simulink model "suspension_controller_road_condition2"  (R2020a)
settings: Solver=VariableStepAuto  StartTime=0.0  StopTime=10.0  MaxStep=0.1  RelTol=1e-3
values from neighbouring files (symbols this model uses):
  cfs = 1290    [half_car_parameter.m]
  cft = 1000    [half_car_parameter.m]
  crs = 1620    [half_car_parameter.m]
  crt = 1000    [half_car_parameter.m]
  iyy = 2460    [half_car_parameter.m]
  kfs = 19960    [half_car_parameter.m]
  kft = 175500    [half_car_parameter.m]
  krs = 17500    [half_car_parameter.m]
  krt = 175500    [half_car_parameter.m]
  lf = 2.3    [half_car_parameter.m]
  lr = 2.3    [half_car_parameter.m]
  mc = 700    [half_car_parameter.m]
  mf = 40    [half_car_parameter.m]
  mr = 35.5    [half_car_parameter.m]
(part 1 of 2)
settings Model: Creator=USER  LastModifiedBy=USER

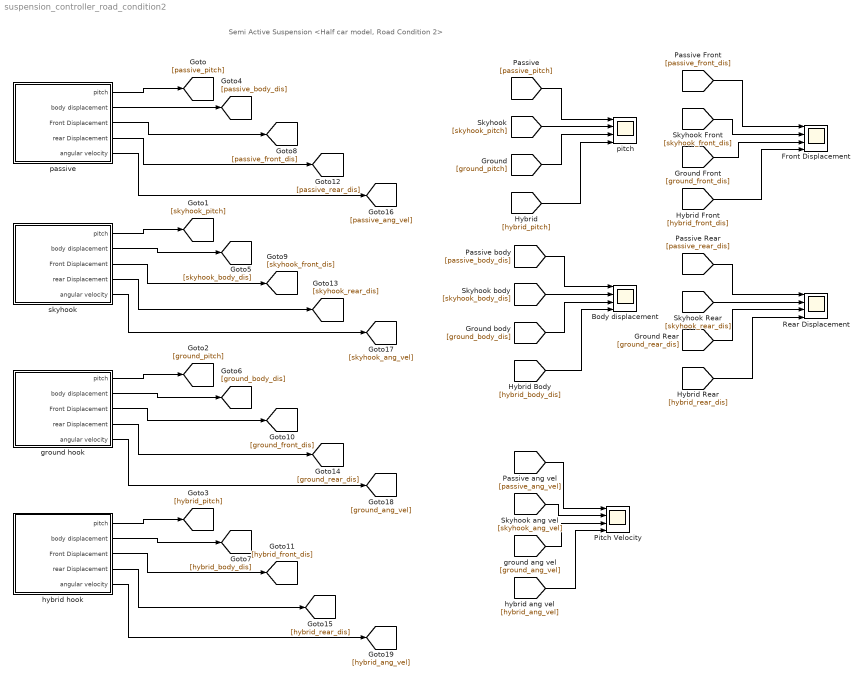
== system suspension_controller_road_condition2 ==
  note: Semi Active Suspension <Half car model, Road Condition 2>
  Body displacement : Scope  NumInputPorts=4
  Front Displacement : Scope  NumInputPorts=4
  Pitch Velocity : Scope  NumInputPorts=4
  Rear Displacement : Scope  NumInputPorts=4
  ground hook : Subsystem
  hybrid hook : Subsystem
  passive : Subsystem
  pitch : Scope  NumInputPorts=4
  skyhook : Subsystem
  wires:
  passive/1(pitch) -> [passive_pitch]
  skyhook/1(pitch) -> [skyhook_pitch]
  ground hook/1(pitch) -> [ground_pitch]
  hybrid hook/1(pitch) -> [hybrid_pitch]
  passive/2(body displacement) -> [passive_body_dis]
  skyhook/2(body displacement) -> [skyhook_body_dis]
  ground hook/2(body displacement) -> [ground_body_dis]
  hybrid hook/2(body displacement) -> [hybrid_body_dis]
  [passive_pitch] -> pitch/1
  [skyhook_pitch] -> pitch/2
  [ground_pitch] -> pitch/3
  [hybrid_pitch] -> pitch/4
  [passive_body_dis] -> Body displacement/1
  [skyhook_body_dis] -> Body displacement/2
  [ground_body_dis] -> Body displacement/3
  [hybrid_body_dis] -> Body displacement/4
  passive/3(Front Displacement) -> [passive_front_dis]
  skyhook/3(Front Displacement) -> [skyhook_front_dis]
  ground hook/3(Front Displacement) -> [ground_front_dis]
  hybrid hook/3(Front Displacement) -> [hybrid_front_dis]
  [passive_front_dis] -> Front Displacement/1
  [skyhook_front_dis] -> Front Displacement/2
  [ground_front_dis] -> Front Displacement/3
  [hybrid_front_dis] -> Front Displacement/4
  passive/4(rear Displacement) -> [passive_rear_dis]
  skyhook/4(rear Displacement) -> [skyhook_rear_dis]
  ground hook/4(rear Displacement) -> [ground_rear_dis]
  hybrid hook/4(rear Displacement) -> [hybrid_rear_dis]
  [hybrid_rear_dis] -> Rear Displacement/4
  [passive_rear_dis] -> Rear Displacement/1
  [ground_rear_dis] -> Rear Displacement/3
  [skyhook_rear_dis] -> Rear Displacement/2
  passive/5(angular velocity) -> [passive_ang_vel]
  skyhook/5(angular velocity) -> [skyhook_ang_vel]
  ground hook/5(angular velocity) -> [ground_ang_vel]
  hybrid hook/5(angular velocity) -> [hybrid_ang_vel]
  [passive_ang_vel] -> Pitch Velocity/1
  [skyhook_ang_vel] -> Pitch Velocity/2
  [ground_ang_vel] -> Pitch Velocity/3
  [hybrid_ang_vel] -> Pitch Velocity/4

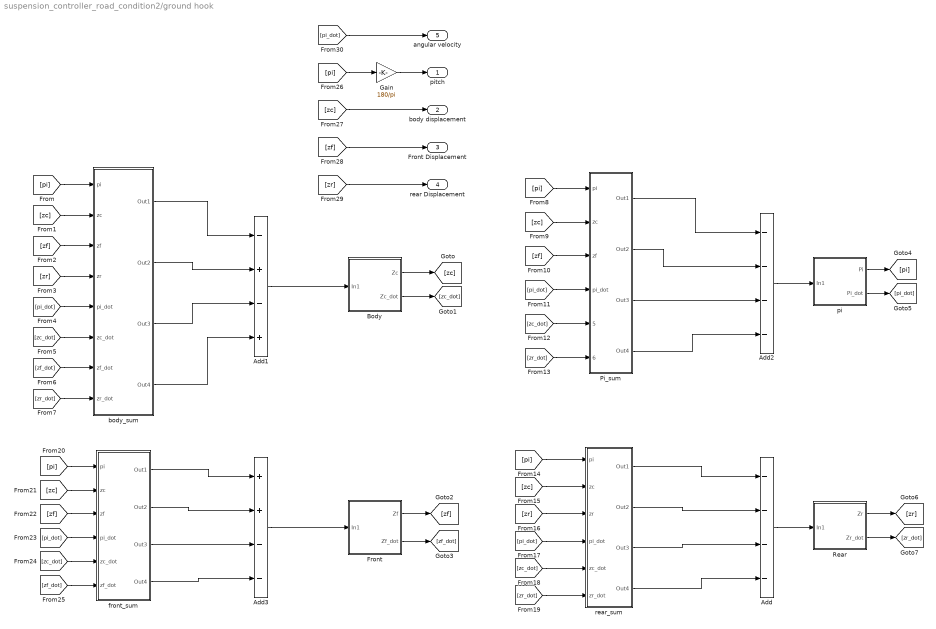
== system suspension_controller_road_condition2/ground hook ==
  Add : Sum  Inputs=----
  Add1 : Sum  Inputs=-+-+
  Add2 : Sum  Inputs=----
  Add3 : Sum  Inputs=++--
  Body : Subsystem
  Front : Subsystem
  Gain : Gain  Gain=180/pi
  Pi_sum : Subsystem
  Rear : Subsystem
  body_sum : Subsystem
  front_sum : Subsystem
  pi : Subsystem
  rear_sum : Subsystem
  pitch : Outport
  body displacement : Outport  Port=2
  Front Displacement : Outport  Port=3
  rear Displacement : Outport  Port=4
  angular velocity : Outport  Port=5
  wires:
  Rear/2(Zr_dot) -> [zr_dot]
  [zc_dot] -> front_sum/5(zc_dot)
  [zr] -> body_sum/4(zr)
  [zr_dot] -> rear_sum/6(zr_dot)
  [pi_dot] -> body_sum/5(pi_dot)
  body_sum/3(Out3) -> Add1/3
  [zr] -> rear_sum/3(zr)
  [pi] -> front_sum/1(pi)
  [zc_dot] -> body_sum/6(zc_dot)
  [zr_dot] -> body_sum/8(zr_dot)
  Front/1(Zf) -> [zf]
  [zf_dot] -> body_sum/7(zf_dot)
  rear_sum/3(Out3) -> Add/3
  body_sum/1(Out1) -> Add1/1
  rear_sum/4(Out4) -> Add/4
  [pi_dot] -> rear_sum/4(pi_dot)
  rear_sum/2(Out2) -> Add/2
  [zc] -> rear_sum/2(zc)
  [pi] -> rear_sum/1(pi)
  Add3/1 -> Front/1(In1)
  rear_sum/1(Out1) -> Add/1
  front_sum/3(Out3) -> Add3/3
  front_sum/4(Out4) -> Add3/4
  front_sum/1(Out1) -> Add3/1
  body_sum/4(Out4) -> Add1/4
  body_sum/2(Out2) -> Add1/2
  Body/1(Zc) -> [zc]
  front_sum/2(Out2) -> Add3/2
  Body/2(Zc_dot) -> [zc_dot]
  Add1/1 -> Body/1(In1)
  Add/1 -> Rear/1(In1)
  [zc] -> body_sum/2(zc)
  [zf] -> body_sum/3(zf)
  [zc_dot] -> rear_sum/5(zc_dot)
  [zf_dot] -> front_sum/6(zf_dot)
  Front/2(Zf_dot) -> [zf_dot]
  Rear/1(Zr) -> [zr]
  [pi] -> body_sum/1(pi)
  [pi_dot] -> front_sum/4(pi_dot)
  [zf] -> front_sum/3(zf)
  [zc] -> front_sum/2(zc)
  Pi_sum/2(Out2) -> Add2/2
  [zc_dot] -> Pi_sum/5(zc_dot)
  [zf] -> Pi_sum/3(zf)
  Pi_sum/4(Out4) -> Add2/4
  [pi] -> Pi_sum/1(pi)
  Pi_sum/3(Out3) -> Add2/3
  [zr_dot] -> Pi_sum/6(zr_dot)
  pi/2(Pi_dot) -> [pi_dot]
  [zc] -> Pi_sum/2(zc)
  [pi_dot] -> Pi_sum/4(pi_dot)
  Pi_sum/1(Out1) -> Add2/1
  pi/1(Pi) -> [pi]
  Add2/1 -> pi/1(In1)
  Gain/1 -> pitch/1
  [pi] -> Gain/1
  [zf] -> Front Displacement/1
  [pi_dot] -> angular velocity/1
  [zr] -> rear Displacement/1
  [zc] -> body displacement/1

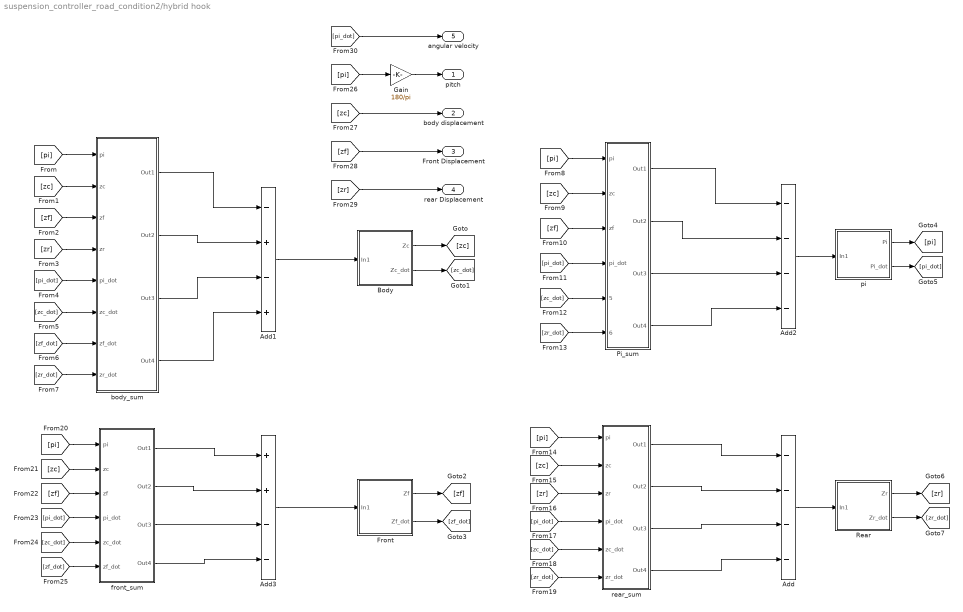
== system suspension_controller_road_condition2/hybrid hook ==
  Add : Sum  Inputs=----
  Add1 : Sum  Inputs=-+-+
  Add2 : Sum  Inputs=----
  Add3 : Sum  Inputs=++--
  Body : Subsystem
  Front : Subsystem
  Gain : Gain  Gain=180/pi
  Pi_sum : Subsystem
  Rear : Subsystem
  body_sum : Subsystem
  front_sum : Subsystem
  pi : Subsystem
  rear_sum : Subsystem
  pitch : Outport
  body displacement : Outport  Port=2
  Front Displacement : Outport  Port=3
  rear Displacement : Outport  Port=4
  angular velocity : Outport  Port=5
  wires:
  Rear/2(Zr_dot) -> [zr_dot]
  [zc_dot] -> front_sum/5(zc_dot)
  [zr] -> body_sum/4(zr)
  [zr_dot] -> rear_sum/6(zr_dot)
  [pi_dot] -> body_sum/5(pi_dot)
  body_sum/3(Out3) -> Add1/3
  [zr] -> rear_sum/3(zr)
  [pi] -> front_sum/1(pi)
  [zc_dot] -> body_sum/6(zc_dot)
  [zr_dot] -> body_sum/8(zr_dot)
  Front/1(Zf) -> [zf]
  [zf_dot] -> body_sum/7(zf_dot)
  rear_sum/3(Out3) -> Add/3
  body_sum/1(Out1) -> Add1/1
  rear_sum/4(Out4) -> Add/4
  [pi_dot] -> rear_sum/4(pi_dot)
  rear_sum/2(Out2) -> Add/2
  [zc] -> rear_sum/2(zc)
  [pi] -> rear_sum/1(pi)
  Add3/1 -> Front/1(In1)
  rear_sum/1(Out1) -> Add/1
  front_sum/3(Out3) -> Add3/3
  front_sum/4(Out4) -> Add3/4
  front_sum/1(Out1) -> Add3/1
  body_sum/4(Out4) -> Add1/4
  body_sum/2(Out2) -> Add1/2
  Body/1(Zc) -> [zc]
  front_sum/2(Out2) -> Add3/2
  Body/2(Zc_dot) -> [zc_dot]
  Add1/1 -> Body/1(In1)
  Add/1 -> Rear/1(In1)
  [zc] -> body_sum/2(zc)
  [zf] -> body_sum/3(zf)
  [zc_dot] -> rear_sum/5(zc_dot)
  [zf_dot] -> front_sum/6(zf_dot)
  Front/2(Zf_dot) -> [zf_dot]
  Rear/1(Zr) -> [zr]
  [pi] -> body_sum/1(pi)
  [pi_dot] -> front_sum/4(pi_dot)
  [zf] -> front_sum/3(zf)
  [zc] -> front_sum/2(zc)
  Pi_sum/2(Out2) -> Add2/2
  [zc_dot] -> Pi_sum/5(zc_dot)
  [zf] -> Pi_sum/3(zf)
  Pi_sum/4(Out4) -> Add2/4
  [pi] -> Pi_sum/1(pi)
  Pi_sum/3(Out3) -> Add2/3
  [zr_dot] -> Pi_sum/6(zr_dot)
  pi/2(Pi_dot) -> [pi_dot]
  [zc] -> Pi_sum/2(zc)
  [pi_dot] -> Pi_sum/4(pi_dot)
  Pi_sum/1(Out1) -> Add2/1
  pi/1(Pi) -> [pi]
  Add2/1 -> pi/1(In1)
  Gain/1 -> pitch/1
  [pi] -> Gain/1
  [zf] -> Front Displacement/1
  [pi_dot] -> angular velocity/1
  [zr] -> rear Displacement/1
  [zc] -> body displacement/1

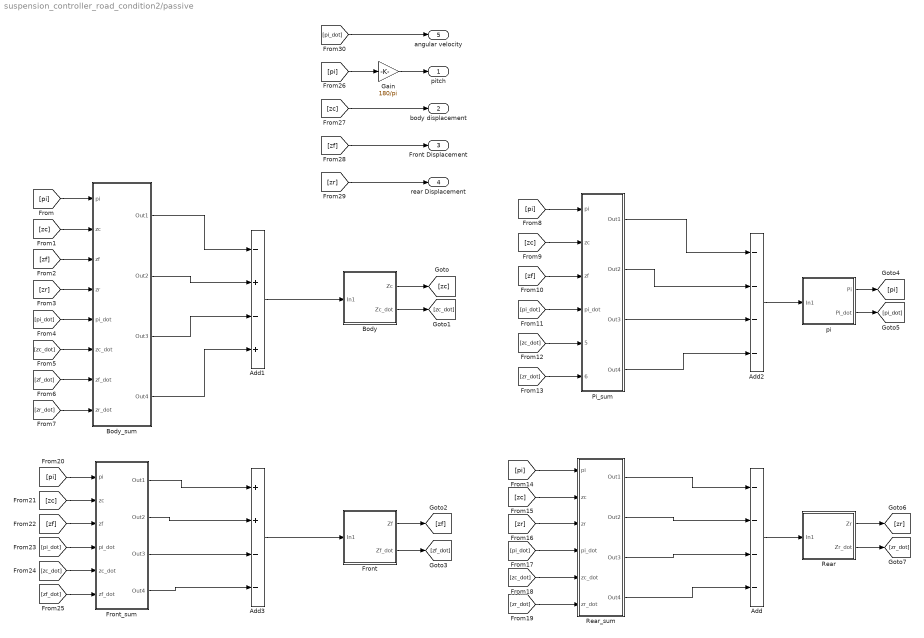
== system suspension_controller_road_condition2/passive ==
  Add : Sum  Inputs=----
  Add1 : Sum  Inputs=-+-+
  Add2 : Sum  Inputs=----
  Add3 : Sum  Inputs=++--
  Body : Subsystem
  Body_sum : Subsystem
  Front : Subsystem
  Front_sum : Subsystem
  Gain : Gain  Gain=180/pi
  Pi_sum : Subsystem
  Rear : Subsystem
  Rear_sum : Subsystem
  pi : Subsystem
  pitch : Outport
  body displacement : Outport  Port=2
  Front Displacement : Outport  Port=3
  rear Displacement : Outport  Port=4
  angular velocity : Outport  Port=5
  wires:
  [zc] -> body displacement/1
  Rear/2(Zr_dot) -> [zr_dot]
  [zc_dot] -> Front_sum/5(zc_dot)
  [zr] -> Body_sum/4(zr)
  [zr_dot] -> Rear_sum/6(zr_dot)
  [pi_dot] -> Body_sum/5(pi_dot)
  Body_sum/3(Out3) -> Add1/3
  [zr] -> Rear_sum/3(zr)
  [pi] -> Front_sum/1(pi)
  [zc_dot] -> Body_sum/6(zc_dot)
  [zr_dot] -> Body_sum/8(zr_dot)
  Front/1(Zf) -> [zf]
  Pi_sum/3(Out3) -> Add2/3
  Pi_sum/2(Out2) -> Add2/2
  [pi] -> Gain/1
  pi/1(Pi) -> [pi]
  [zf_dot] -> Body_sum/7(zf_dot)
  Rear_sum/3(Out3) -> Add/3
  Body_sum/1(Out1) -> Add1/1
  Rear_sum/4(Out4) -> Add/4
  [zc_dot] -> Pi_sum/5(zc_dot)
  [pi_dot] -> Rear_sum/4(pi_dot)
  [zr_dot] -> Pi_sum/6(zr_dot)
  Rear_sum/2(Out2) -> Add/2
  [zc] -> Pi_sum/2(zc)
  [zc] -> Rear_sum/2(zc)
  [pi] -> Rear_sum/1(pi)
  Add3/1 -> Front/1(In1)
  Rear_sum/1(Out1) -> Add/1
  Front_sum/3(Out3) -> Add3/3
  Front_sum/4(Out4) -> Add3/4
  [pi] -> Pi_sum/1(pi)
  Add2/1 -> pi/1(In1)
  Front_sum/1(Out1) -> Add3/1
  Pi_sum/4(Out4) -> Add2/4
  Pi_sum/1(Out1) -> Add2/1
  Body_sum/4(Out4) -> Add1/4
  Body_sum/2(Out2) -> Add1/2
  Body/1(Zc) -> [zc]
  [pi_dot] -> Pi_sum/4(pi_dot)
  Front_sum/2(Out2) -> Add3/2
  Body/2(Zc_dot) -> [zc_dot]
  Add1/1 -> Body/1(In1)
  Add/1 -> Rear/1(In1)
  pi/2(Pi_dot) -> [pi_dot]
  [zc] -> Body_sum/2(zc)
  [zf] -> Body_sum/3(zf)
  [zc_dot] -> Rear_sum/5(zc_dot)
  [zf_dot] -> Front_sum/6(zf_dot)
  Front/2(Zf_dot) -> [zf_dot]
  Rear/1(Zr) -> [zr]
  [pi] -> Body_sum/1(pi)
  [pi_dot] -> Front_sum/4(pi_dot)
  [zf] -> Front_sum/3(zf)
  [zf] -> Pi_sum/3(zf)
  [zc] -> Front_sum/2(zc)
  Gain/1 -> pitch/1
  [zf] -> Front Displacement/1
  [zr] -> rear Displacement/1
  [pi_dot] -> angular velocity/1

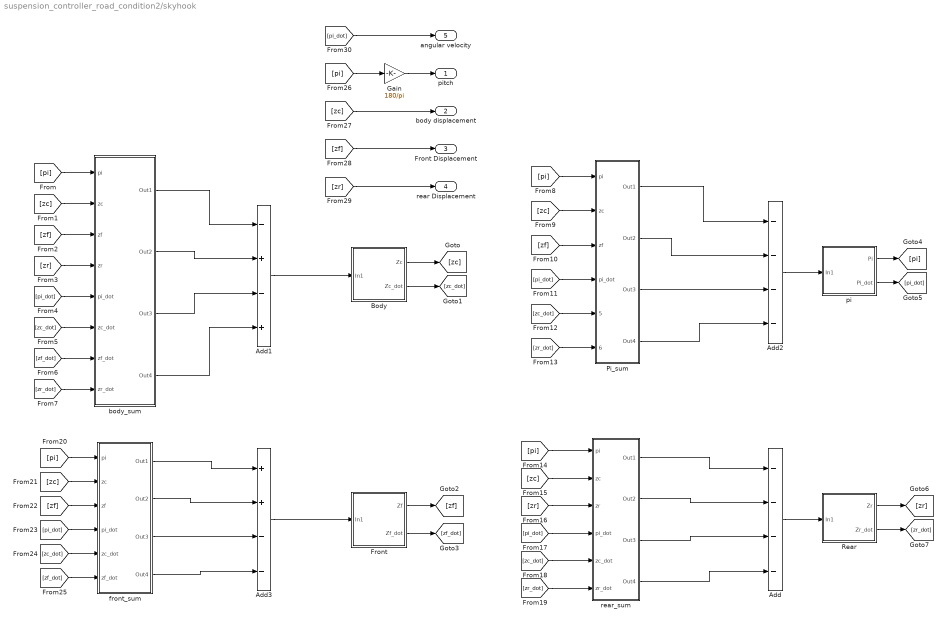
== system suspension_controller_road_condition2/skyhook ==
  Add : Sum  Inputs=----
  Add1 : Sum  Inputs=-+-+
  Add2 : Sum  Inputs=----
  Add3 : Sum  Inputs=++--
  Body : Subsystem
  Front : Subsystem
  Gain : Gain  Gain=180/pi
  Pi_sum : Subsystem
  Rear : Subsystem
  body_sum : Subsystem
  front_sum : Subsystem
  pi : Subsystem
  rear_sum : Subsystem
  pitch : Outport
  body displacement : Outport  Port=2
  Front Displacement : Outport  Port=3
  rear Displacement : Outport  Port=4
  angular velocity : Outport  Port=5
  wires:
  Rear/2(Zr_dot) -> [zr_dot]
  [zc_dot] -> front_sum/5(zc_dot)
  [zr] -> body_sum/4(zr)
  [zr_dot] -> rear_sum/6(zr_dot)
  [pi_dot] -> body_sum/5(pi_dot)
  body_sum/3(Out3) -> Add1/3
  [zr] -> rear_sum/3(zr)
  [pi] -> front_sum/1(pi)
  [zc_dot] -> body_sum/6(zc_dot)
  [zr_dot] -> body_sum/8(zr_dot)
  Front/1(Zf) -> [zf]
  [zf_dot] -> body_sum/7(zf_dot)
  rear_sum/3(Out3) -> Add/3
  body_sum/1(Out1) -> Add1/1
  rear_sum/4(Out4) -> Add/4
  [pi_dot] -> rear_sum/4(pi_dot)
  rear_sum/2(Out2) -> Add/2
  [zc] -> rear_sum/2(zc)
  [pi] -> rear_sum/1(pi)
  Add3/1 -> Front/1(In1)
  rear_sum/1(Out1) -> Add/1
  front_sum/3(Out3) -> Add3/3
  front_sum/4(Out4) -> Add3/4
  front_sum/1(Out1) -> Add3/1
  body_sum/4(Out4) -> Add1/4
  body_sum/2(Out2) -> Add1/2
  Body/1(Zc) -> [zc]
  front_sum/2(Out2) -> Add3/2
  Body/2(Zc_dot) -> [zc_dot]
  Add1/1 -> Body/1(In1)
  Add/1 -> Rear/1(In1)
  [zc] -> body_sum/2(zc)
  [zf] -> body_sum/3(zf)
  [zc_dot] -> rear_sum/5(zc_dot)
  [zf_dot] -> front_sum/6(zf_dot)
  Front/2(Zf_dot) -> [zf_dot]
  Rear/1(Zr) -> [zr]
  [pi] -> body_sum/1(pi)
  [pi_dot] -> front_sum/4(pi_dot)
  [zf] -> front_sum/3(zf)
  [zc] -> front_sum/2(zc)
  Pi_sum/2(Out2) -> Add2/2
  [zc_dot] -> Pi_sum/5(zc_dot)
  [zf] -> Pi_sum/3(zf)
  Pi_sum/4(Out4) -> Add2/4
  [pi] -> Pi_sum/1(pi)
  Pi_sum/3(Out3) -> Add2/3
  [zr_dot] -> Pi_sum/6(zr_dot)
  pi/2(Pi_dot) -> [pi_dot]
  [zc] -> Pi_sum/2(zc)
  [pi_dot] -> Pi_sum/4(pi_dot)
  Pi_sum/1(Out1) -> Add2/1
  pi/1(Pi) -> [pi]
  Add2/1 -> pi/1(In1)
  Gain/1 -> pitch/1
  [pi] -> Gain/1
  [zf] -> Front Displacement/1
  [pi_dot] -> angular velocity/1
  [zr] -> rear Displacement/1
  [zc] -> body displacement/1

== system suspension_controller_road_condition2/ground hook/Body ==
  In1 : Inport
  Gain1 : Gain  Gain=1/mc
  zc : Integrator
  zc_dot : Integrator
  Zc : Outport
  Zc_dot : Outport  Port=2
  wires:
  Gain1/1 -> zc_dot/1  "zc_ddot"
  zc_dot/1 -> Zc_dot/1, zc/1
  In1/1 -> Gain1/1
  zc/1 -> Zc/1

== system suspension_controller_road_condition2/ground hook/Front ==
  In1 : Inport
  Gain2 : Gain  Gain=1/mf
  zf : Integrator
  zf_dot : Integrator
  Zf : Outport
  Zf_dot : Outport  Port=2
  wires:
  In1/1 -> Gain2/1
  zf_dot/1 -> Zf_dot/1, zf/1
  Gain2/1 -> zf_dot/1  "zf_ddot"
  zf/1 -> Zf/1

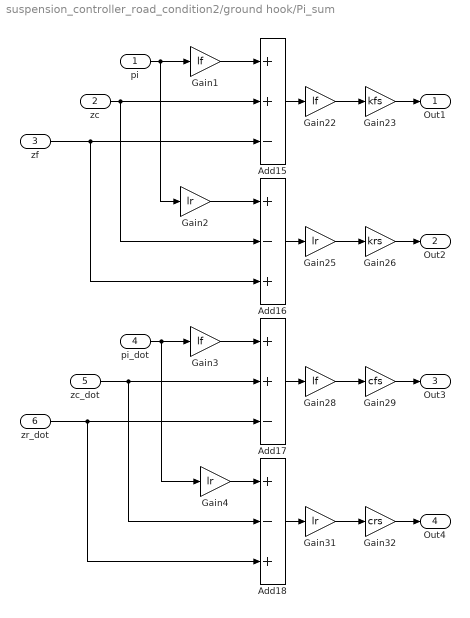
== system suspension_controller_road_condition2/ground hook/Pi_sum ==
  pi : Inport
  zc : Inport  Port=2
  zf : Inport  Port=3
  pi_dot : Inport  Port=4
  zc_dot : Inport  Port=5
  zr_dot : Inport  Port=6
  Add15 : Sum  Inputs=++-
  Add16 : Sum  Inputs=+-+
  Add17 : Sum  Inputs=++-
  Add18 : Sum  Inputs=+-+
  Gain{1,3,22,28} (4 alike) : Gain  Gain=lf
  Gain{2,4,25,31} (4 alike) : Gain  Gain=lr
  Gain23 : Gain  Gain=kfs
  Gain26 : Gain  Gain=krs
  Gain29 : Gain  Gain=cfs
  Gain32 : Gain  Gain=crs
  Out1 : Outport
  Out2 : Outport  Port=2
  Out3 : Outport  Port=3
  Out4 : Outport  Port=4
  wires:
  pi/1 -> Gain2/1, Gain1/1
  Add16/1 -> Gain25/1
  zc_dot/1 -> Add18/2, Add17/2
  zc/1 -> Add15/2, Add16/2
  Add17/1 -> Gain28/1
  zf/1 -> Add16/3, Add15/3
  Add15/1 -> Gain22/1
  pi_dot/1 -> Gain4/1, Gain3/1
  zr_dot/1 -> Add18/3, Add17/3
  Add18/1 -> Gain31/1
  Gain22/1 -> Gain23/1
  Gain23/1 -> Out1/1
  Gain25/1 -> Gain26/1
  Gain26/1 -> Out2/1
  Gain28/1 -> Gain29/1
  Gain29/1 -> Out3/1
  Gain31/1 -> Gain32/1
  Gain32/1 -> Out4/1
  Gain1/1 -> Add15/1
  Gain2/1 -> Add16/1
  Gain3/1 -> Add17/1
  Gain4/1 -> Add18/1

== system suspension_controller_road_condition2/ground hook/Rear ==
  In1 : Inport
  Gain2 : Gain  Gain=1/mr
  zr : Integrator
  zr_dot : Integrator
  Zr : Outport
  Zr_dot : Outport  Port=2
  wires:
  In1/1 -> Gain2/1
  zr_dot/1 -> Zr_dot/1, zr/1
  Gain2/1 -> zr_dot/1  "zr_ddot"
  zr/1 -> Zr/1

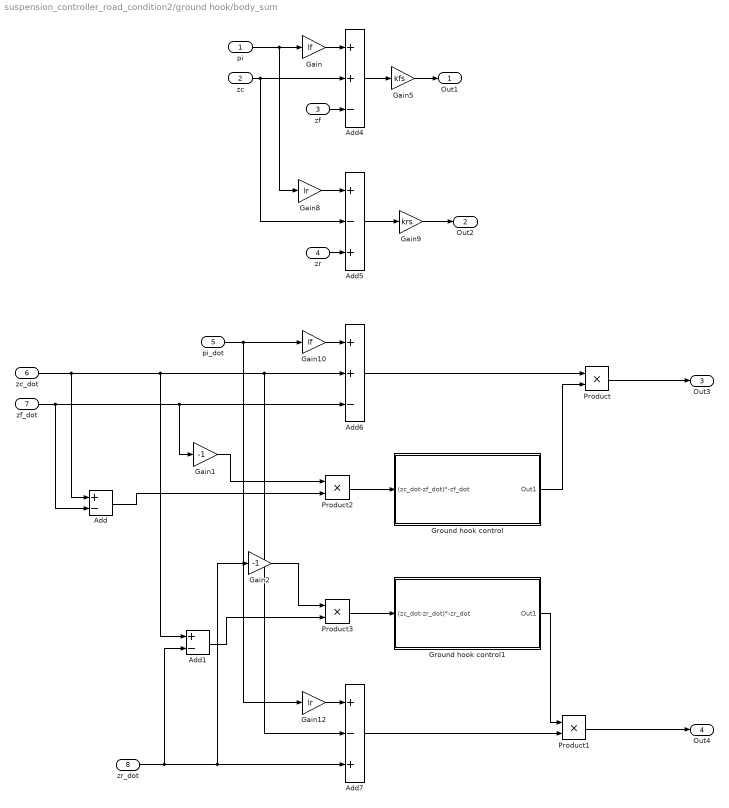
== system suspension_controller_road_condition2/ground hook/body_sum ==
  pi : Inport
  zc : Inport  Port=2
  zf : Inport  Port=3
  zr : Inport  Port=4
  pi_dot : Inport  Port=5
  zc_dot : Inport  Port=6
  zf_dot : Inport  Port=7
  zr_dot : Inport  Port=8
  Add : Sum  Inputs=+-
  Add1 : Sum  Inputs=+-
  Add4 : Sum  Inputs=++-
  Add5 : Sum  Inputs=+-+
  Add6 : Sum  Inputs=++-
  Add7 : Sum  Inputs=+-+
  Gain : Gain  Gain=lf
  Gain1 : Gain  Gain=-1
  Gain10 : Gain  Gain=lf
  Gain12 : Gain  Gain=lr
  Gain2 : Gain  Gain=-1
  Gain5 : Gain  Gain=kfs
  Gain8 : Gain  Gain=lr
  Gain9 : Gain  Gain=krs
  Ground hook control : Subsystem
  Ground hook control1 : Subsystem
  Product{,1..3} (4 alike) : Product
  Out1 : Outport
  Out2 : Outport  Port=2
  Out3 : Outport  Port=3
  Out4 : Outport  Port=4
  wires:
  zf/1 -> Add4/3
  Add7/1 -> Product1/2
  zr_dot/1 -> Add1/2, Gain2/1, Add7/3
  zc/1 -> Add4/2, Add5/2
  zc_dot/1 -> Add1/1, Add7/2, Add6/2, Add/1
  Add4/1 -> Gain5/1
  zr/1 -> Add5/3
  pi_dot/1 -> Gain10/1, Gain12/1
  pi/1 -> Gain8/1, Gain/1
  Add6/1 -> Product/1
  zf_dot/1 -> Gain1/1, Add6/3, Add/2
  Add5/1 -> Gain9/1
  Gain/1 -> Add4/1
  Gain8/1 -> Add5/1
  Gain5/1 -> Out1/1
  Gain9/1 -> Out2/1
  Gain10/1 -> Add6/1
  Product/1 -> Out3/1
  Gain12/1 -> Add7/1
  Product1/1 -> Out4/1
  Add/1 -> Product2/2
  Add1/1 -> Product3/2
  Gain1/1 -> Product2/1
  Product2/1 -> Ground hook control/1((zc_dot-zf_dot)*-zf_dot)
  Ground hook control/1(Out1) -> Product/2
  Gain2/1 -> Product3/1
  Product3/1 -> Ground hook control1/1((zc_dot-zr_dot)*-zr_dot)
  Ground hook control1/1(Out1) -> Product1/1

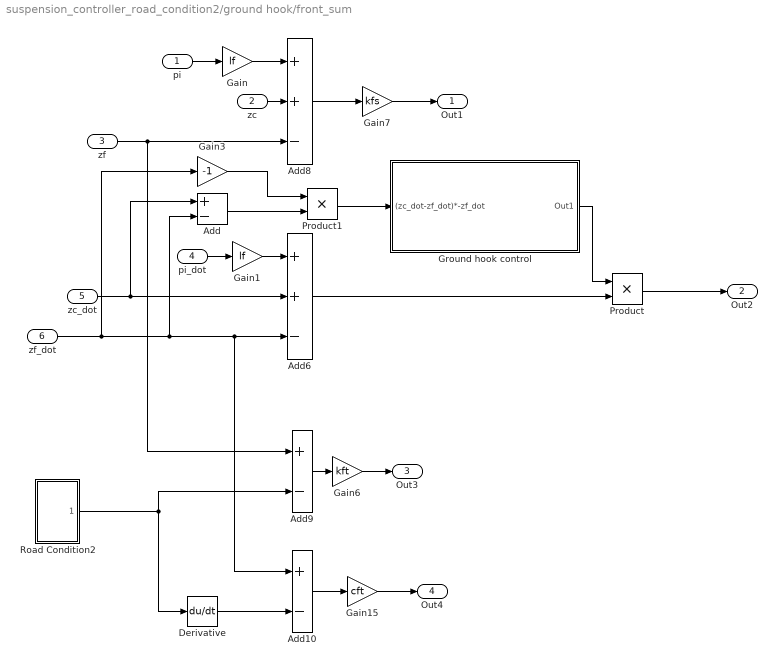
== system suspension_controller_road_condition2/ground hook/front_sum ==
  pi : Inport
  zc : Inport  Port=2
  zf : Inport  Port=3
  pi_dot : Inport  Port=4
  zc_dot : Inport  Port=5
  zf_dot : Inport  Port=6
  Add : Sum  Inputs=+-
  Add10 : Sum  Inputs=+-
  Add6 : Sum  Inputs=++-
  Add8 : Sum  Inputs=++-
  Add9 : Sum  Inputs=+-
  Derivative : Derivative
  Gain : Gain  Gain=lf
  Gain1 : Gain  Gain=lf
  Gain15 : Gain  Gain=cft
  Gain3 : Gain  Gain=-1
  Gain6 : Gain  Gain=kft
  Gain7 : Gain  Gain=kfs
  Ground hook control : Subsystem
  Product : Product
  Product1 : Product
  Road Condition2 : Subsystem
  Out1 : Outport
  Out2 : Outport  Port=2
  Out3 : Outport  Port=3
  Out4 : Outport  Port=4
  wires:
  Add8/1 -> Gain7/1
  zc_dot/1 -> Add/1, Add6/2
  zf_dot/1 -> Gain3/1, Add/2, Add6/3, Add10/1
  zf/1 -> Add8/3, Add9/1
  pi_dot/1 -> Gain1/1
  zc/1 -> Add8/2
  Add9/1 -> Gain6/1
  pi/1 -> Gain/1
  Add6/1 -> Product/2
  Derivative/1 -> Add10/2
  Add10/1 -> Gain15/1
  Gain7/1 -> Out1/1
  Product/1 -> Out2/1
  Gain6/1 -> Out3/1
  Gain15/1 -> Out4/1
  Gain/1 -> Add8/1
  Gain1/1 -> Add6/1
  Add/1 -> Product1/2
  Gain3/1 -> Product1/1
  Product1/1 -> Ground hook control/1((zc_dot-zf_dot)*-zf_dot)
  Ground hook control/1(Out1) -> Product/1
  Road Condition2/1(Output) -> Derivative/1, Add9/2

== system suspension_controller_road_condition2/ground hook/pi ==
  In1 : Inport
  Gain2 : Gain  Gain=1/iyy
  pi : Integrator
  pi_dot : Integrator
  Pi : Outport
  Pi_dot : Outport  Port=2
  wires:
  In1/1 -> Gain2/1
  pi_dot/1 -> Pi_dot/1, pi/1
  Gain2/1 -> pi_dot/1  "pi_ddot"
  pi/1 -> Pi/1

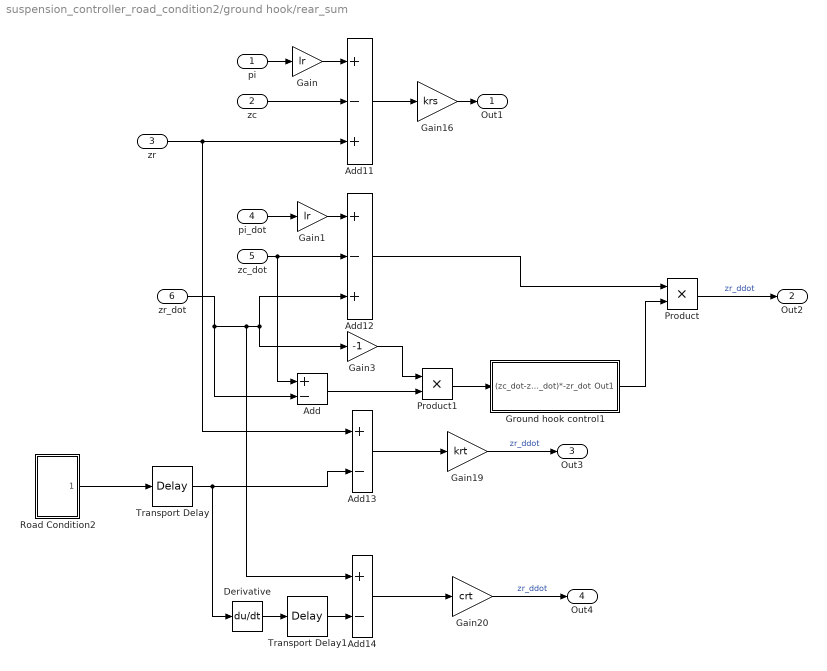
== system suspension_controller_road_condition2/ground hook/rear_sum ==
  pi : Inport
  zc : Inport  Port=2
  zr : Inport  Port=3
  pi_dot : Inport  Port=4
  zc_dot : Inport  Port=5
  zr_dot : Inport  Port=6
  Add : Sum  Inputs=+-
  Add11 : Sum  Inputs=+-+
  Add12 : Sum  Inputs=+-+
  Add13 : Sum  Inputs=+-
  Add14 : Sum  Inputs=+-
  Derivative : Derivative
  Gain : Gain  Gain=lr
  Gain1 : Gain  Gain=lr
  Gain16 : Gain  Gain=krs
  Gain19 : Gain  Gain=krt
  Gain20 : Gain  Gain=crt
  Gain3 : Gain  Gain=-1
  Ground hook control1 : Subsystem
  Product : Product
  Product1 : Product
  Road Condition2 : Subsystem
  Transport Delay : TransportDelay  DelayTime=0.3
  Transport Delay1 : TransportDelay  DelayTime=0.3
  Out1 : Outport
  Out2 : Outport  Port=2
  Out3 : Outport  Port=3
  Out4 : Outport  Port=4
  wires:
  Add14/1 -> Gain20/1
  zr_dot/1 -> Add/2, Gain3/1, Add12/3, Add14/1
  pi_dot/1 -> Gain1/1
  Transport Delay1/1 -> Add14/2
  Add13/1 -> Gain19/1
  zc/1 -> Add11/2
  Add12/1 -> Product/1
  zr/1 -> Add13/1, Add11/3
  zc_dot/1 -> Add/1, Add12/2
  Add11/1 -> Gain16/1
  pi/1 -> Gain/1
  Gain16/1 -> Out1/1
  Product/1 -> Out2/1  "zr_ddot"
  Gain19/1 -> Out3/1  "zr_ddot"
  Gain20/1 -> Out4/1  "zr_ddot"
  Gain/1 -> Add11/1
  Gain1/1 -> Add12/1
  Transport Delay/1 -> Derivative/1, Add13/2
  Derivative/1 -> Transport Delay1/1
  Add/1 -> Product1/2
  Gain3/1 -> Product1/1
  Product1/1 -> Ground hook control1/1((zc_dot-zr_dot)*-zr_dot)
  Ground hook control1/1(Out1) -> Product/2
  Road Condition2/1(Output) -> Transport Delay/1

== system suspension_controller_road_condition2/hybrid hook/Body ==
  In1 : Inport
  Gain1 : Gain  Gain=1/mc
  zc : Integrator
  zc_dot : Integrator
  Zc : Outport
  Zc_dot : Outport  Port=2
  wires:
  Gain1/1 -> zc_dot/1  "zc_ddot"
  zc_dot/1 -> Zc_dot/1, zc/1
  In1/1 -> Gain1/1
  zc/1 -> Zc/1

== system suspension_controller_road_condition2/hybrid hook/Front ==
  In1 : Inport
  Gain2 : Gain  Gain=1/mf
  zf : Integrator
  zf_dot : Integrator
  Zf : Outport
  Zf_dot : Outport  Port=2
  wires:
  In1/1 -> Gain2/1
  zf_dot/1 -> Zf_dot/1, zf/1
  Gain2/1 -> zf_dot/1  "zf_ddot"
  zf/1 -> Zf/1

== system suspension_controller_road_condition2/hybrid hook/Pi_sum ==
  pi : Inport
  zc : Inport  Port=2
  zf : Inport  Port=3
  pi_dot : Inport  Port=4
  zc_dot : Inport  Port=5
  zr_dot : Inport  Port=6
  Add15 : Sum  Inputs=++-
  Add16 : Sum  Inputs=+-+
  Add17 : Sum  Inputs=++-
  Add18 : Sum  Inputs=+-+
  Gain{1,3,22,28} (4 alike) : Gain  Gain=lf
  Gain{2,4,25,31} (4 alike) : Gain  Gain=lr
  Gain23 : Gain  Gain=kfs
  Gain26 : Gain  Gain=krs
  Gain29 : Gain  Gain=cfs
  Gain32 : Gain  Gain=crs
  Out1 : Outport
  Out2 : Outport  Port=2
  Out3 : Outport  Port=3
  Out4 : Outport  Port=4
  wires:
  pi/1 -> Gain2/1, Gain1/1
  Add16/1 -> Gain25/1
  zc_dot/1 -> Add18/2, Add17/2
  zc/1 -> Add15/2, Add16/2
  Add17/1 -> Gain28/1
  zf/1 -> Add16/3, Add15/3
  Add15/1 -> Gain22/1
  pi_dot/1 -> Gain4/1, Gain3/1
  zr_dot/1 -> Add18/3, Add17/3
  Add18/1 -> Gain31/1
  Gain22/1 -> Gain23/1
  Gain23/1 -> Out1/1
  Gain25/1 -> Gain26/1
  Gain26/1 -> Out2/1
  Gain28/1 -> Gain29/1
  Gain29/1 -> Out3/1
  Gain31/1 -> Gain32/1
  Gain32/1 -> Out4/1
  Gain1/1 -> Add15/1
  Gain2/1 -> Add16/1
  Gain3/1 -> Add17/1
  Gain4/1 -> Add18/1

== system suspension_controller_road_condition2/hybrid hook/Rear ==
  In1 : Inport
  Gain2 : Gain  Gain=1/mr
  zr : Integrator
  zr_dot : Integrator
  Zr : Outport
  Zr_dot : Outport  Port=2
  wires:
  In1/1 -> Gain2/1
  zr_dot/1 -> Zr_dot/1, zr/1
  Gain2/1 -> zr_dot/1  "zr_ddot"
  zr/1 -> Zr/1

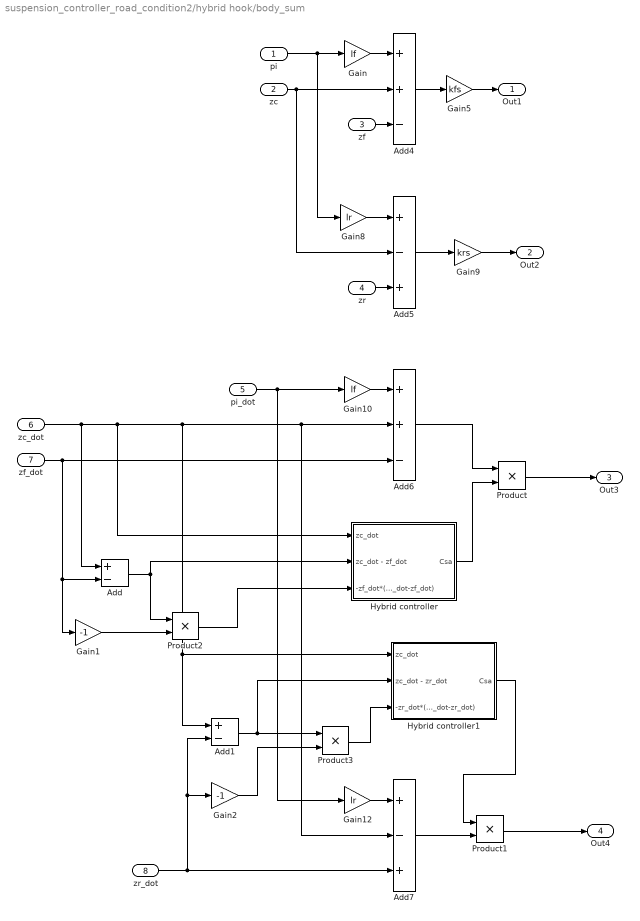
== system suspension_controller_road_condition2/hybrid hook/body_sum ==
  pi : Inport
  zc : Inport  Port=2
  zf : Inport  Port=3
  zr : Inport  Port=4
  pi_dot : Inport  Port=5
  zc_dot : Inport  Port=6
  zf_dot : Inport  Port=7
  zr_dot : Inport  Port=8
  Add : Sum  Inputs=+-
  Add1 : Sum  Inputs=+-
  Add4 : Sum  Inputs=++-
  Add5 : Sum  Inputs=+-+
  Add6 : Sum  Inputs=++-
  Add7 : Sum  Inputs=+-+
  Gain : Gain  Gain=lf
  Gain1 : Gain  Gain=-1
  Gain10 : Gain  Gain=lf
  Gain12 : Gain  Gain=lr
  Gain2 : Gain  Gain=-1
  Gain5 : Gain  Gain=kfs
  Gain8 : Gain  Gain=lr
  Gain9 : Gain  Gain=krs
  Hybrid controller : Subsystem
  Hybrid controller1 : Subsystem
  Product{,1..3} (4 alike) : Product
  Out1 : Outport
  Out2 : Outport  Port=2
  Out3 : Outport  Port=3
  Out4 : Outport  Port=4
  wires:
  zf/1 -> Add4/3
  Add7/1 -> Product1/2
  zr_dot/1 -> Gain2/1, Add1/2, Add7/3
  zc/1 -> Add4/2, Add5/2
  zc_dot/1 -> Hybrid controller/1(zc_dot), Add1/1, Hybrid controller1/1(zc_dot), Add7/2, Add6/2, Add/1
  Add4/1 -> Gain5/1
  zr/1 -> Add5/3
  pi_dot/1 -> Gain10/1, Gain12/1
  pi/1 -> Gain8/1, Gain/1
  Add6/1 -> Product/1
  zf_dot/1 -> Add6/3, Gain1/1, Add/2
  Add5/1 -> Gain9/1
  Gain/1 -> Add4/1
  Gain8/1 -> Add5/1
  Gain5/1 -> Out1/1
  Gain9/1 -> Out2/1
  Gain10/1 -> Add6/1
  Product/1 -> Out3/1
  Gain12/1 -> Add7/1
  Product1/1 -> Out4/1
  Add/1 -> Product2/1, Hybrid controller/2(zc_dot - zf_dot)
  Add1/1 -> Product3/1, Hybrid controller1/2(zc_dot - zr_dot)
  Gain1/1 -> Product2/2
  Product2/1 -> Hybrid controller/3(-zf_dot*(zc_dot-zf_dot))
  Hybrid controller/1(Csa) -> Product/2
  Gain2/1 -> Product3/2
  Product3/1 -> Hybrid controller1/3(-zr_dot*(zc_dot-zr_dot))
  Hybrid controller1/1(Csa) -> Product1/1

== system suspension_controller_road_condition2/hybrid hook/front_sum ==
  pi : Inport
  zc : Inport  Port=2
  zf : Inport  Port=3
  pi_dot : Inport  Port=4
  zc_dot : Inport  Port=5
  zf_dot : Inport  Port=6
  Add : Sum  Inputs=+-
  Add10 : Sum  Inputs=+-
  Add6 : Sum  Inputs=++-
  Add8 : Sum  Inputs=++-
  Add9 : Sum  Inputs=+-
  Derivative : Derivative
  Gain : Gain  Gain=lf
  Gain1 : Gain  Gain=lf
  Gain15 : Gain  Gain=cft
  Gain3 : Gain  Gain=-1
  Gain6 : Gain  Gain=kft
  Gain7 : Gain  Gain=kfs
  Hybrid controller : Subsystem
  Product : Product
  Product1 : Product
  Road Condition2 : Subsystem
  Out1 : Outport
  Out2 : Outport  Port=2
  Out3 : Outport  Port=3
  Out4 : Outport  Port=4
  wires:
  Add8/1 -> Gain7/1
  zc_dot/1 -> Hybrid controller/1(zc_dot), Add/1, Add6/2
  zf_dot/1 -> Gain3/1, Add/2, Add6/3, Add10/1
  zf/1 -> Add8/3, Add9/1
  pi_dot/1 -> Gain1/1
  zc/1 -> Add8/2
  Add9/1 -> Gain6/1
  pi/1 -> Gain/1
  Add6/1 -> Product/2
  Derivative/1 -> Add10/2
  Add10/1 -> Gain15/1
  Gain7/1 -> Out1/1
  Product/1 -> Out2/1
  Gain6/1 -> Out3/1
  Gain15/1 -> Out4/1
  Gain/1 -> Add8/1
  Gain1/1 -> Add6/1
  Add/1 -> Hybrid controller/2(zc_dot - zf_dot), Product1/2
  Gain3/1 -> Product1/1
  Product1/1 -> Hybrid controller/3(-zf_dot*(zc_dot-zf_dot))
  Hybrid controller/1(Csa) -> Product/1
  Road Condition2/1(Output) -> Derivative/1, Add9/2

== system suspension_controller_road_condition2/hybrid hook/pi ==
  In1 : Inport
  Gain2 : Gain  Gain=1/iyy
  pi : Integrator
  pi_dot : Integrator
  Pi : Outport
  Pi_dot : Outport  Port=2
  wires:
  In1/1 -> Gain2/1
  pi_dot/1 -> Pi_dot/1, pi/1
  Gain2/1 -> pi_dot/1  "pi_ddot"
  pi/1 -> Pi/1

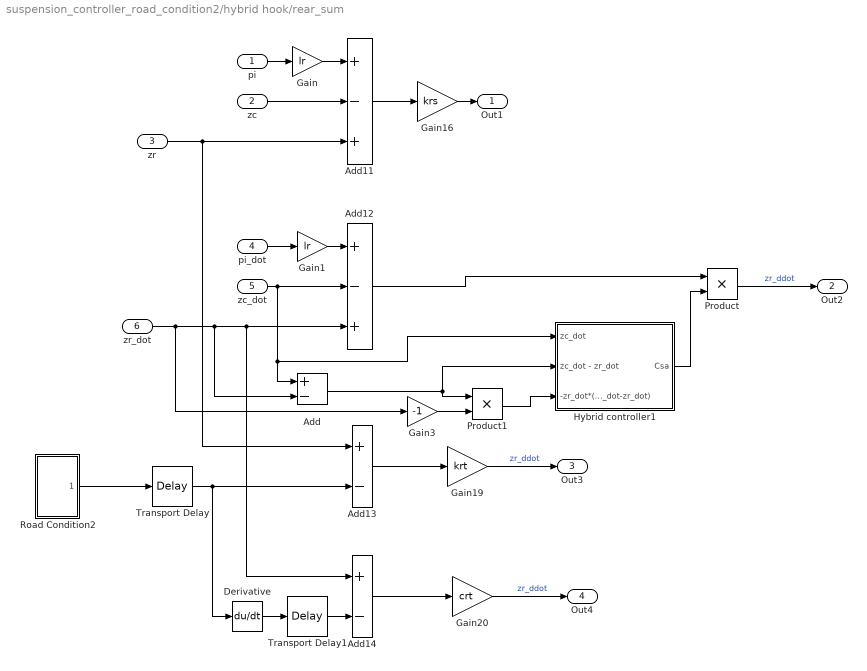
== system suspension_controller_road_condition2/hybrid hook/rear_sum ==
  pi : Inport
  zc : Inport  Port=2
  zr : Inport  Port=3
  pi_dot : Inport  Port=4
  zc_dot : Inport  Port=5
  zr_dot : Inport  Port=6
  Add : Sum  Inputs=+-
  Add11 : Sum  Inputs=+-+
  Add12 : Sum  Inputs=+-+
  Add13 : Sum  Inputs=+-
  Add14 : Sum  Inputs=+-
  Derivative : Derivative
  Gain : Gain  Gain=lr
  Gain1 : Gain  Gain=lr
  Gain16 : Gain  Gain=krs
  Gain19 : Gain  Gain=krt
  Gain20 : Gain  Gain=crt
  Gain3 : Gain  Gain=-1
  Hybrid controller1 : Subsystem
  Product : Product
  Product1 : Product
  Road Condition2 : Subsystem
  Transport Delay : TransportDelay  DelayTime=0.3
  Transport Delay1 : TransportDelay  DelayTime=0.3
  Out1 : Outport
  Out2 : Outport  Port=2
  Out3 : Outport  Port=3
  Out4 : Outport  Port=4
  wires:
  Add14/1 -> Gain20/1
  zr_dot/1 -> Gain3/1, Add/2, Add12/3, Add14/1
  pi_dot/1 -> Gain1/1
  Transport Delay1/1 -> Add14/2
  Add13/1 -> Gain19/1
  zc/1 -> Add11/2
  Add12/1 -> Product/1
  zr/1 -> Add13/1, Add11/3
  zc_dot/1 -> Add12/2, Hybrid controller1/1(zc_dot), Add/1
  Add11/1 -> Gain16/1
  pi/1 -> Gain/1
  Gain16/1 -> Out1/1
  Product/1 -> Out2/1  "zr_ddot"
  Gain19/1 -> Out3/1  "zr_ddot"
  Gain20/1 -> Out4/1  "zr_ddot"
  Gain/1 -> Add11/1
  Gain1/1 -> Add12/1
  Transport Delay/1 -> Derivative/1, Add13/2
  Derivative/1 -> Transport Delay1/1
  Add/1 -> Product1/1, Hybrid controller1/2(zc_dot - zr_dot)
  Gain3/1 -> Product1/2
  Product1/1 -> Hybrid controller1/3(-zr_dot*(zc_dot-zr_dot))
  Hybrid controller1/1(Csa) -> Product/2
  Road Condition2/1(Output) -> Transport Delay/1

== system suspension_controller_road_condition2/passive/Body ==
  In1 : Inport
  Gain1 : Gain  Gain=1/mc
  zc : Integrator
  zc_dot : Integrator
  Zc : Outport
  Zc_dot : Outport  Port=2
  wires:
  Gain1/1 -> zc_dot/1  "zc_ddot"
  zc_dot/1 -> Zc_dot/1, zc/1
  In1/1 -> Gain1/1
  zc/1 -> Zc/1

== system suspension_controller_road_condition2/passive/Body_sum ==
  pi : Inport
  zc : Inport  Port=2
  zf : Inport  Port=3
  zr : Inport  Port=4
  pi_dot : Inport  Port=5
  zc_dot : Inport  Port=6
  zf_dot : Inport  Port=7
  zr_dot : Inport  Port=8
  Add4 : Sum  Inputs=++-
  Add5 : Sum  Inputs=+-+
  Add6 : Sum  Inputs=++-
  Add7 : Sum  Inputs=+-+
  Gain : Gain  Gain=lf
  Gain10 : Gain  Gain=lf
  Gain11 : Gain  Gain=cfs
  Gain12 : Gain  Gain=lr
  Gain13 : Gain  Gain=crs
  Gain5 : Gain  Gain=kfs
  Gain8 : Gain  Gain=lr
  Gain9 : Gain  Gain=krs
  Out1 : Outport
  Out2 : Outport  Port=2
  Out3 : Outport  Port=3
  Out4 : Outport  Port=4
  wires:
  zf/1 -> Add4/3
  Add7/1 -> Gain13/1
  zr_dot/1 -> Add7/3
  zc/1 -> Add4/2, Add5/2
  zc_dot/1 -> Add7/2, Add6/2
  Add4/1 -> Gain5/1
  zr/1 -> Add5/3
  pi_dot/1 -> Gain10/1, Gain12/1
  pi/1 -> Gain8/1, Gain/1
  Add6/1 -> Gain11/1
  zf_dot/1 -> Add6/3
  Add5/1 -> Gain9/1
  Gain/1 -> Add4/1
  Gain8/1 -> Add5/1
  Gain5/1 -> Out1/1
  Gain9/1 -> Out2/1
  Gain10/1 -> Add6/1
  Gain11/1 -> Out3/1
  Gain12/1 -> Add7/1
  Gain13/1 -> Out4/1

== system suspension_controller_road_condition2/passive/Front ==
  In1 : Inport
  Gain2 : Gain  Gain=1/mf
  zf : Integrator
  zf_dot : Integrator
  Zf : Outport
  Zf_dot : Outport  Port=2
  wires:
  In1/1 -> Gain2/1
  zf_dot/1 -> Zf_dot/1, zf/1
  Gain2/1 -> zf_dot/1  "zf_ddot"
  zf/1 -> Zf/1

== system suspension_controller_road_condition2/passive/Front_sum ==
  pi : Inport
  zc : Inport  Port=2
  zf : Inport  Port=3
  pi_dot : Inport  Port=4
  zc_dot : Inport  Port=5
  zf_dot : Inport  Port=6
  Add10 : Sum  Inputs=+-
  Add6 : Sum  Inputs=++-
  Add8 : Sum  Inputs=++-
  Add9 : Sum  Inputs=+-
  Derivative : Derivative
  Gain : Gain  Gain=lf
  Gain1 : Gain  Gain=lf
  Gain11 : Gain  Gain=cfs
  Gain15 : Gain  Gain=cft
  Gain6 : Gain  Gain=kft
  Gain7 : Gain  Gain=kfs
  Road Condition2 : Subsystem
  Out1 : Outport
  Out2 : Outport  Port=2
  Out3 : Outport  Port=3
  Out4 : Outport  Port=4
  wires:
  Add8/1 -> Gain7/1
  zc_dot/1 -> Add6/2
  zf_dot/1 -> Add6/3, Add10/1
  zf/1 -> Add8/3, Add9/1
  pi_dot/1 -> Gain1/1
  zc/1 -> Add8/2
  Add9/1 -> Gain6/1
  pi/1 -> Gain/1
  Add6/1 -> Gain11/1
  Derivative/1 -> Add10/2
  Add10/1 -> Gain15/1
  Gain7/1 -> Out1/1
  Gain11/1 -> Out2/1
  Gain6/1 -> Out3/1
  Gain15/1 -> Out4/1
  Gain/1 -> Add8/1
  Gain1/1 -> Add6/1
  Road Condition2/1(Output) -> Derivative/1, Add9/2

== system suspension_controller_road_condition2/passive/Pi_sum ==
  pi : Inport
  zc : Inport  Port=2
  zf : Inport  Port=3
  pi_dot : Inport  Port=4
  zc_dot : Inport  Port=5
  zr_dot : Inport  Port=6
  Add15 : Sum  Inputs=++-
  Add16 : Sum  Inputs=+-+
  Add17 : Sum  Inputs=++-
  Add18 : Sum  Inputs=+-+
  Gain{1,3,22,28} (4 alike) : Gain  Gain=lf
  Gain{2,4,25,31} (4 alike) : Gain  Gain=lr
  Gain23 : Gain  Gain=kfs
  Gain26 : Gain  Gain=krs
  Gain29 : Gain  Gain=cfs
  Gain32 : Gain  Gain=crs
  Out1 : Outport
  Out2 : Outport  Port=2
  Out3 : Outport  Port=3
  Out4 : Outport  Port=4
  wires:
  pi/1 -> Gain2/1, Gain1/1
  Add16/1 -> Gain25/1
  zc_dot/1 -> Add18/2, Add17/2
  zc/1 -> Add15/2, Add16/2
  Add17/1 -> Gain28/1
  zf/1 -> Add16/3, Add15/3
  Add15/1 -> Gain22/1
  pi_dot/1 -> Gain4/1, Gain3/1
  zr_dot/1 -> Add18/3, Add17/3
  Add18/1 -> Gain31/1
  Gain22/1 -> Gain23/1
  Gain23/1 -> Out1/1
  Gain25/1 -> Gain26/1
  Gain26/1 -> Out2/1
  Gain28/1 -> Gain29/1
  Gain29/1 -> Out3/1
  Gain31/1 -> Gain32/1
  Gain32/1 -> Out4/1
  Gain1/1 -> Add15/1
  Gain2/1 -> Add16/1
  Gain3/1 -> Add17/1
  Gain4/1 -> Add18/1

== system suspension_controller_road_condition2/passive/Rear ==
  In1 : Inport
  Gain2 : Gain  Gain=1/mr
  zr : Integrator
  zr_dot : Integrator
  Zr : Outport
  Zr_dot : Outport  Port=2
  wires:
  In1/1 -> Gain2/1
  zr_dot/1 -> Zr_dot/1, zr/1
  Gain2/1 -> zr_dot/1  "zr_ddot"
  zr/1 -> Zr/1

== system suspension_controller_road_condition2/passive/Rear_sum ==
  pi : Inport
  zc : Inport  Port=2
  zr : Inport  Port=3
  pi_dot : Inport  Port=4
  zc_dot : Inport  Port=5
  zr_dot : Inport  Port=6
  Add11 : Sum  Inputs=+-+
  Add12 : Sum  Inputs=+-+
  Add13 : Sum  Inputs=+-
  Add14 : Sum  Inputs=+-
  Derivative : Derivative
  Gain : Gain  Gain=lr
  Gain1 : Gain  Gain=lr
  Gain16 : Gain  Gain=krs
  Gain18 : Gain  Gain=crs
  Gain19 : Gain  Gain=krt
  Gain20 : Gain  Gain=crt
  Road Condition2 : Subsystem
  Transport Delay : TransportDelay  DelayTime=0.3
  Transport Delay1 : TransportDelay  DelayTime=0.3
  Out1 : Outport
  Out2 : Outport  Port=2
  Out3 : Outport  Port=3
  Out4 : Outport  Port=4
  wires:
  Add14/1 -> Gain20/1
  zr_dot/1 -> Add12/3, Add14/1
  pi_dot/1 -> Gain1/1
  Transport Delay1/1 -> Add14/2
  Add13/1 -> Gain19/1
  zc/1 -> Add11/2
  Add12/1 -> Gain18/1
  zr/1 -> Add13/1, Add11/3
  zc_dot/1 -> Add12/2
  Add11/1 -> Gain16/1
  pi/1 -> Gain/1
  Gain16/1 -> Out1/1
  Gain18/1 -> Out2/1  "zr_ddot"
  Gain19/1 -> Out3/1  "zr_ddot"
  Gain20/1 -> Out4/1  "zr_ddot"
  Gain/1 -> Add11/1
  Gain1/1 -> Add12/1
  Transport Delay/1 -> Derivative/1, Add13/2
  Derivative/1 -> Transport Delay1/1
  Road Condition2/1(Output) -> Transport Delay/1

== system suspension_controller_road_condition2/passive/pi ==
  In1 : Inport
  Gain2 : Gain  Gain=1/iyy
  pi : Integrator
  pi_dot : Integrator
  Pi : Outport
  Pi_dot : Outport  Port=2
  wires:
  In1/1 -> Gain2/1
  pi_dot/1 -> Pi_dot/1, pi/1
  Gain2/1 -> pi_dot/1  "pi_ddot"
  pi/1 -> Pi/1

== system suspension_controller_road_condition2/skyhook/Body ==
  In1 : Inport
  Gain1 : Gain  Gain=1/mc
  zc : Integrator
  zc_dot : Integrator
  Zc : Outport
  Zc_dot : Outport  Port=2
  wires:
  Gain1/1 -> zc_dot/1  "zc_ddot"
  zc_dot/1 -> Zc_dot/1, zc/1
  In1/1 -> Gain1/1
  zc/1 -> Zc/1

== system suspension_controller_road_condition2/skyhook/Front ==
  In1 : Inport
  Gain2 : Gain  Gain=1/mf
  zf : Integrator
  zf_dot : Integrator
  Zf : Outport
  Zf_dot : Outport  Port=2
  wires:
  In1/1 -> Gain2/1
  zf_dot/1 -> Zf_dot/1, zf/1
  Gain2/1 -> zf_dot/1  "zf_ddot"
  zf/1 -> Zf/1

== system suspension_controller_road_condition2/skyhook/Pi_sum ==
  pi : Inport
  zc : Inport  Port=2
  zf : Inport  Port=3
  pi_dot : Inport  Port=4
  zc_dot : Inport  Port=5
  zr_dot : Inport  Port=6
  Add15 : Sum  Inputs=++-
  Add16 : Sum  Inputs=+-+
  Add17 : Sum  Inputs=++-
  Add18 : Sum  Inputs=+-+
  Gain{1,3,22,28} (4 alike) : Gain  Gain=lf
  Gain{2,4,25,31} (4 alike) : Gain  Gain=lr
  Gain23 : Gain  Gain=kfs
  Gain26 : Gain  Gain=krs
  Gain29 : Gain  Gain=cfs
  Gain32 : Gain  Gain=crs
  Out1 : Outport
  Out2 : Outport  Port=2
  Out3 : Outport  Port=3
  Out4 : Outport  Port=4
  wires:
  pi/1 -> Gain2/1, Gain1/1
  Add16/1 -> Gain25/1
  zc_dot/1 -> Add18/2, Add17/2
  zc/1 -> Add15/2, Add16/2
  Add17/1 -> Gain28/1
  zf/1 -> Add16/3, Add15/3
  Add15/1 -> Gain22/1
  pi_dot/1 -> Gain4/1, Gain3/1
  zr_dot/1 -> Add18/3, Add17/3
  Add18/1 -> Gain31/1
  Gain22/1 -> Gain23/1
  Gain23/1 -> Out1/1
  Gain25/1 -> Gain26/1
  Gain26/1 -> Out2/1
  Gain28/1 -> Gain29/1
  Gain29/1 -> Out3/1
  Gain31/1 -> Gain32/1
  Gain32/1 -> Out4/1
  Gain1/1 -> Add15/1
  Gain2/1 -> Add16/1
  Gain3/1 -> Add17/1
  Gain4/1 -> Add18/1

== system suspension_controller_road_condition2/skyhook/Rear ==
  In1 : Inport
  Gain2 : Gain  Gain=1/mr
  zr : Integrator
  zr_dot : Integrator
  Zr : Outport
  Zr_dot : Outport  Port=2
  wires:
  In1/1 -> Gain2/1
  zr_dot/1 -> Zr_dot/1, zr/1
  Gain2/1 -> zr_dot/1  "zr_ddot"
  zr/1 -> Zr/1

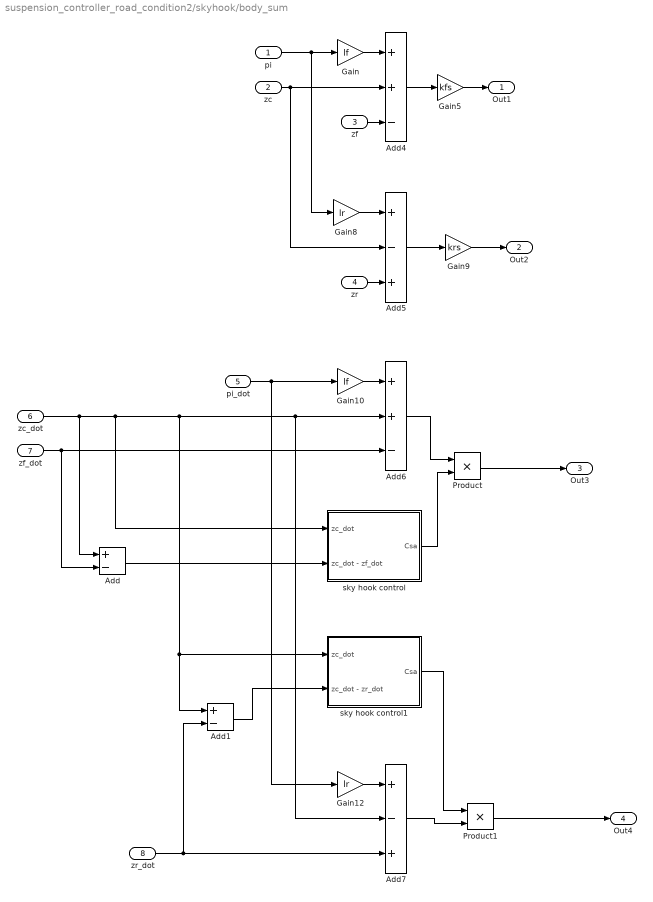
== system suspension_controller_road_condition2/skyhook/body_sum ==
  pi : Inport
  zc : Inport  Port=2
  zf : Inport  Port=3
  zr : Inport  Port=4
  pi_dot : Inport  Port=5
  zc_dot : Inport  Port=6
  zf_dot : Inport  Port=7
  zr_dot : Inport  Port=8
  Add : Sum  Inputs=+-
  Add1 : Sum  Inputs=+-
  Add4 : Sum  Inputs=++-
  Add5 : Sum  Inputs=+-+
  Add6 : Sum  Inputs=++-
  Add7 : Sum  Inputs=+-+
  Gain : Gain  Gain=lf
  Gain10 : Gain  Gain=lf
  Gain12 : Gain  Gain=lr
  Gain5 : Gain  Gain=kfs
  Gain8 : Gain  Gain=lr
  Gain9 : Gain  Gain=krs
  Product : Product
  Product1 : Product
  sky hook control : Subsystem
  sky hook control1 : Subsystem
  Out1 : Outport
  Out2 : Outport  Port=2
  Out3 : Outport  Port=3
  Out4 : Outport  Port=4
  wires:
  zf/1 -> Add4/3
  Add7/1 -> Product1/2
  zr_dot/1 -> Add1/2, Add7/3
  zc/1 -> Add4/2, Add5/2
  zc_dot/1 -> sky hook control/1(zc_dot), Add1/1, sky hook control1/1(zc_dot), Add7/2, Add6/2, Add/1
  Add4/1 -> Gain5/1
  zr/1 -> Add5/3
  pi_dot/1 -> Gain10/1, Gain12/1
  pi/1 -> Gain8/1, Gain/1
  Add6/1 -> Product/1
  zf_dot/1 -> Add6/3, Add/2
  Add5/1 -> Gain9/1
  Gain/1 -> Add4/1
  Gain8/1 -> Add5/1
  Gain5/1 -> Out1/1
  Gain9/1 -> Out2/1
  Gain10/1 -> Add6/1
  Product/1 -> Out3/1
  Gain12/1 -> Add7/1
  Product1/1 -> Out4/1
  Add/1 -> sky hook control/2(zc_dot - zf_dot)
  sky hook control/1(Csa) -> Product/2
  Add1/1 -> sky hook control1/2(zc_dot - zr_dot)
  sky hook control1/1(Csa) -> Product1/1

== system suspension_controller_road_condition2/skyhook/front_sum ==
  pi : Inport
  zc : Inport  Port=2
  zf : Inport  Port=3
  pi_dot : Inport  Port=4
  zc_dot : Inport  Port=5
  zf_dot : Inport  Port=6
  Add : Sum  Inputs=+-
  Add10 : Sum  Inputs=+-
  Add6 : Sum  Inputs=++-
  Add8 : Sum  Inputs=++-
  Add9 : Sum  Inputs=+-
  Derivative : Derivative
  Gain : Gain  Gain=lf
  Gain1 : Gain  Gain=lf
  Gain15 : Gain  Gain=cft
  Gain6 : Gain  Gain=kft
  Gain7 : Gain  Gain=kfs
  Product : Product
  Road Condition2 : Subsystem
  sky hook control : Subsystem
  Out1 : Outport
  Out2 : Outport  Port=2
  Out3 : Outport  Port=3
  Out4 : Outport  Port=4
  wires:
  Add8/1 -> Gain7/1
  zc_dot/1 -> Add/1, sky hook control/1(zc_dot), Add6/2
  zf_dot/1 -> Add/2, Add6/3, Add10/1
  zf/1 -> Add8/3, Add9/1
  pi_dot/1 -> Gain1/1
  zc/1 -> Add8/2
  Add9/1 -> Gain6/1
  pi/1 -> Gain/1
  Add6/1 -> Product/2
  Derivative/1 -> Add10/2
  Add10/1 -> Gain15/1
  Gain7/1 -> Out1/1
  Product/1 -> Out2/1
  Gain6/1 -> Out3/1
  Gain15/1 -> Out4/1
  Gain/1 -> Add8/1
  Gain1/1 -> Add6/1
  Add/1 -> sky hook control/2(zc_dot - zf_dot)
  sky hook control/1(Csa) -> Product/1
  Road Condition2/1(Output) -> Derivative/1, Add9/2

== system suspension_controller_road_condition2/skyhook/pi ==
  In1 : Inport
  Gain2 : Gain  Gain=1/iyy
  pi : Integrator
  pi_dot : Integrator
  Pi : Outport
  Pi_dot : Outport  Port=2
  wires:
  In1/1 -> Gain2/1
  pi_dot/1 -> Pi_dot/1, pi/1
  Gain2/1 -> pi_dot/1  "pi_ddot"
  pi/1 -> Pi/1

== system suspension_controller_road_condition2/skyhook/rear_sum ==
  pi : Inport
  zc : Inport  Port=2
  zr : Inport  Port=3
  pi_dot : Inport  Port=4
  zc_dot : Inport  Port=5
  zr_dot : Inport  Port=6
  Add : Sum  Inputs=+-
  Add11 : Sum  Inputs=+-+
  Add12 : Sum  Inputs=+-+
  Add13 : Sum  Inputs=+-
  Add14 : Sum  Inputs=+-
  Derivative : Derivative
  Gain : Gain  Gain=lr
  Gain1 : Gain  Gain=lr
  Gain16 : Gain  Gain=krs
  Gain19 : Gain  Gain=krt
  Gain20 : Gain  Gain=crt
  Product : Product
  Road Condition2 : Subsystem
  Transport Delay : TransportDelay  DelayTime=0.3
  Transport Delay1 : TransportDelay  DelayTime=0.3
  sky hook control : Subsystem
  Out1 : Outport
  Out2 : Outport  Port=2
  Out3 : Outport  Port=3
  Out4 : Outport  Port=4
  wires:
  Add14/1 -> Gain20/1
  zr_dot/1 -> Add/2, Add12/3, Add14/1
  pi_dot/1 -> Gain1/1
  Transport Delay1/1 -> Add14/2
  Add13/1 -> Gain19/1
  zc/1 -> Add11/2
  Add12/1 -> Product/1
  zr/1 -> Add13/1, Add11/3
  zc_dot/1 -> Add12/2, sky hook control/1(zc_dot), Add/1
  Add11/1 -> Gain16/1
  pi/1 -> Gain/1
  Gain16/1 -> Out1/1
  Product/1 -> Out2/1  "zr_ddot"
  Gain19/1 -> Out3/1  "zr_ddot"
  Gain20/1 -> Out4/1  "zr_ddot"
  Gain/1 -> Add11/1
  Gain1/1 -> Add12/1
  Transport Delay/1 -> Derivative/1, Add13/2
  Derivative/1 -> Transport Delay1/1
  Add/1 -> sky hook control/2(zc_dot - zr_dot)
  sky hook control/1(Csa) -> Product/2
  Road Condition2/1(Output) -> Transport Delay/1

== system suspension_controller_road_condition2/ground hook/body_sum/Ground hook control ==
  (zc_dot-zf_dot)*-zf_dot : Inport
  Constant : Constant  Value=2838
  Constant1 : Constant  Value=258
  If : If  IfExpression=u1 >= 0  ZeroCross=off
  If Action Subsystem : Subsystem  TreatAsAtomicUnit=on
  If Action Subsystem1 : Subsystem  TreatAsAtomicUnit=on
  Merge : Merge
  Out1 : Outport
  wires:
  If/2 -> If Action Subsystem1/Action
  If Action Subsystem1/1(Out1) -> Merge/2
  Constant/1 -> If Action Subsystem/1(In1)
  If/1 -> If Action Subsystem/Action
  (zc_dot-zf_dot)*-zf_dot/1 -> If/1
  If Action Subsystem/1(Csa) -> Merge/1
  Constant1/1 -> If Action Subsystem1/1(In1)
  Merge/1 -> Out1/1

== system suspension_controller_road_condition2/ground hook/body_sum/Ground hook control1 ==
  (zc_dot-zr_dot)*-zr_dot : Inport
  Constant : Constant  Value=2838
  Constant1 : Constant  Value=258
  If : If  IfExpression=u1 >= 0  ZeroCross=off
  If Action Subsystem : Subsystem  TreatAsAtomicUnit=on
  If Action Subsystem1 : Subsystem  TreatAsAtomicUnit=on
  Merge : Merge
  Out1 : Outport
  wires:
  If/2 -> If Action Subsystem1/Action
  If Action Subsystem1/1(Out1) -> Merge/2
  Constant/1 -> If Action Subsystem/1(In1)
  If/1 -> If Action Subsystem/Action
  (zc_dot-zr_dot)*-zr_dot/1 -> If/1
  If Action Subsystem/1(Csa) -> Merge/1
  Constant1/1 -> If Action Subsystem1/1(In1)
  Merge/1 -> Out1/1

== system suspension_controller_road_condition2/ground hook/front_sum/Ground hook control ==
  (zc_dot-zf_dot)*-zf_dot : Inport
  Constant : Constant  Value=2838
  Constant1 : Constant  Value=258
  If : If  IfExpression=u1 >= 0  ZeroCross=off
  If Action Subsystem : Subsystem  TreatAsAtomicUnit=on
  If Action Subsystem1 : Subsystem  TreatAsAtomicUnit=on
  Merge : Merge
  Out1 : Outport
  wires:
  If/2 -> If Action Subsystem1/Action
  If Action Subsystem1/1(Out1) -> Merge/2
  Constant/1 -> If Action Subsystem/1(In1)
  If/1 -> If Action Subsystem/Action
  (zc_dot-zf_dot)*-zf_dot/1 -> If/1
  If Action Subsystem/1(Csa) -> Merge/1
  Constant1/1 -> If Action Subsystem1/1(In1)
  Merge/1 -> Out1/1

== system suspension_controller_road_condition2/ground hook/front_sum/Road Condition2 ==
  Product : Product  Inputs=3
  Saturation : Saturate  LowerLimit=0
  Scope : Scope
  Signal Generator : SignalGenerator  Amplitude=0.15  Frequency=1.852
  Step : Step  SampleTime=1.08
  Step1 : Step  Before=1  After=0  SampleTime=4
  Output : Outport
  wires:
  Signal Generator/1 -> Product/1
  Step/1 -> Product/2
  Step1/1 -> Product/3
  Product/1 -> Output/1, Saturation/1
  Saturation/1 -> Scope/1

== system suspension_controller_road_condition2/ground hook/rear_sum/Ground hook control1 ==
  (zc_dot-zr_dot)*-zr_dot : Inport
  Constant : Constant  Value=2838
  Constant1 : Constant  Value=258
  If : If  IfExpression=u1 >= 0  ZeroCross=off
  If Action Subsystem : Subsystem  TreatAsAtomicUnit=on
  If Action Subsystem1 : Subsystem  TreatAsAtomicUnit=on
  Merge : Merge
  Out1 : Outport
  wires:
  If/2 -> If Action Subsystem1/Action
  If Action Subsystem1/1(Out1) -> Merge/2
  Constant/1 -> If Action Subsystem/1(In1)
  If/1 -> If Action Subsystem/Action
  (zc_dot-zr_dot)*-zr_dot/1 -> If/1
  If Action Subsystem/1(Csa) -> Merge/1
  Constant1/1 -> If Action Subsystem1/1(In1)
  Merge/1 -> Out1/1

== system suspension_controller_road_condition2/ground hook/rear_sum/Road Condition2 ==
  Product : Product  Inputs=3
  Saturation : Saturate  LowerLimit=0
  Scope : Scope
  Signal Generator : SignalGenerator  Amplitude=0.15  Frequency=1.852
  Step : Step  SampleTime=1.08
  Step1 : Step  Before=1  After=0  SampleTime=4
  Output : Outport
  wires:
  Signal Generator/1 -> Product/1
  Step/1 -> Product/2
  Step1/1 -> Product/3
  Product/1 -> Output/1, Saturation/1
  Saturation/1 -> Scope/1

== system suspension_controller_road_condition2/hybrid hook/body_sum/Hybrid controller ==
  zc_dot : Inport
  zc_dot - zf_dot : Inport  Port=2
  -zf_dot*(zc_dot-zf_dot) : Inport  Port=3
  Add : Sum
  Constant : Constant  Value=2838
  Constant1 : Constant  Value=258
  Constant2 : Constant  Value=2838
  Constant3 : Constant  Value=258
  If : If  IfExpression=u1 >= 0  ZeroCross=off
  If Action Subsystem : Subsystem  TreatAsAtomicUnit=on
  If Action Subsystem1 : Subsystem  TreatAsAtomicUnit=on
  If Action Subsystem2 : Subsystem  TreatAsAtomicUnit=on
  If Action Subsystem3 : Subsystem  TreatAsAtomicUnit=on
  If1 : If  IfExpression=u1 >= 0  ZeroCross=off
  Merge : Merge
  Merge1 : Merge
  Product : Product
  Csa : Outport
  wires:
  zc_dot/1 -> Product/1
  Product/1 -> If/1
  If/1 -> If Action Subsystem/Action
  Constant/1 -> If Action Subsystem/1(In1)
  If/2 -> If Action Subsystem1/Action
  If Action Subsystem/1(Csa) -> Merge/1
  If Action Subsystem1/1(Out1) -> Merge/2
  Constant1/1 -> If Action Subsystem1/1(In1)
  zc_dot - zf_dot/1 -> Product/2
  If Action Subsystem2/1(Csa) -> Merge1/1
  If Action Subsystem3/1(Out1) -> Merge1/2
  If1/1 -> If Action Subsystem2/Action
  -zf_dot*(zc_dot-zf_dot)/1 -> If1/1
  Constant2/1 -> If Action Subsystem2/1(In1)
  Constant3/1 -> If Action Subsystem3/1(In1)
  If1/2 -> If Action Subsystem3/Action
  Merge/1 -> Add/1
  Merge1/1 -> Add/2
  Add/1 -> Csa/1

== system suspension_controller_road_condition2/hybrid hook/body_sum/Hybrid controller1 ==
  zc_dot : Inport
  zc_dot - zr_dot : Inport  Port=2
  -zr_dot*(zc_dot-zr_dot) : Inport  Port=3
  Add : Sum
  Constant : Constant  Value=2838
  Constant1 : Constant  Value=258
  Constant2 : Constant  Value=2838
  Constant3 : Constant  Value=258
  If : If  IfExpression=u1 >= 0  ZeroCross=off
  If Action Subsystem : Subsystem  TreatAsAtomicUnit=on
  If Action Subsystem1 : Subsystem  TreatAsAtomicUnit=on
  If Action Subsystem2 : Subsystem  TreatAsAtomicUnit=on
  If Action Subsystem3 : Subsystem  TreatAsAtomicUnit=on
  If1 : If  IfExpression=u1 >= 0  ZeroCross=off
  Merge : Merge
  Merge1 : Merge
  Product : Product
  Csa : Outport
  wires:
  zc_dot/1 -> Product/1
  Product/1 -> If/1
  If/1 -> If Action Subsystem/Action
  Constant/1 -> If Action Subsystem/1(In1)
  If/2 -> If Action Subsystem1/Action
  If Action Subsystem/1(Csa) -> Merge/1
  If Action Subsystem1/1(Out1) -> Merge/2
  Constant1/1 -> If Action Subsystem1/1(In1)
  zc_dot - zr_dot/1 -> Product/2
  If Action Subsystem2/1(Csa) -> Merge1/1
  If Action Subsystem3/1(Out1) -> Merge1/2
  If1/1 -> If Action Subsystem2/Action
  -zr_dot*(zc_dot-zr_dot)/1 -> If1/1
  Constant2/1 -> If Action Subsystem2/1(In1)
  Constant3/1 -> If Action Subsystem3/1(In1)
  If1/2 -> If Action Subsystem3/Action
  Merge/1 -> Add/1
  Merge1/1 -> Add/2
  Add/1 -> Csa/1

== system suspension_controller_road_condition2/hybrid hook/front_sum/Hybrid controller ==
  zc_dot : Inport
  zc_dot - zf_dot : Inport  Port=2
  -zf_dot*(zc_dot-zf_dot) : Inport  Port=3
  Add : Sum
  Constant : Constant  Value=2838
  Constant1 : Constant  Value=258
  Constant2 : Constant  Value=2838
  Constant3 : Constant  Value=258
  If : If  IfExpression=u1 >= 0  ZeroCross=off
  If Action Subsystem : Subsystem  TreatAsAtomicUnit=on
  If Action Subsystem1 : Subsystem  TreatAsAtomicUnit=on
  If Action Subsystem2 : Subsystem  TreatAsAtomicUnit=on
  If Action Subsystem3 : Subsystem  TreatAsAtomicUnit=on
  If1 : If  IfExpression=u1 >= 0  ZeroCross=off
  Merge : Merge
  Merge1 : Merge
  Product : Product
  Csa : Outport
  wires:
  zc_dot/1 -> Product/1
  Product/1 -> If/1
  If/1 -> If Action Subsystem/Action
  Constant/1 -> If Action Subsystem/1(In1)
  If/2 -> If Action Subsystem1/Action
  If Action Subsystem/1(Csa) -> Merge/1
  If Action Subsystem1/1(Out1) -> Merge/2
  Constant1/1 -> If Action Subsystem1/1(In1)
  zc_dot - zf_dot/1 -> Product/2
  If Action Subsystem2/1(Csa) -> Merge1/1
  If Action Subsystem3/1(Out1) -> Merge1/2
  If1/1 -> If Action Subsystem2/Action
  -zf_dot*(zc_dot-zf_dot)/1 -> If1/1
  Constant2/1 -> If Action Subsystem2/1(In1)
  Constant3/1 -> If Action Subsystem3/1(In1)
  If1/2 -> If Action Subsystem3/Action
  Merge/1 -> Add/1
  Merge1/1 -> Add/2
  Add/1 -> Csa/1

== system suspension_controller_road_condition2/hybrid hook/front_sum/Road Condition2 ==
  Product : Product  Inputs=3
  Saturation : Saturate  LowerLimit=0
  Scope : Scope
  Signal Generator : SignalGenerator  Amplitude=0.15  Frequency=1.852
  Step : Step  SampleTime=1.08
  Step1 : Step  Before=1  After=0  SampleTime=4
  Output : Outport
  wires:
  Signal Generator/1 -> Product/1
  Step/1 -> Product/2
  Step1/1 -> Product/3
  Product/1 -> Output/1, Saturation/1
  Saturation/1 -> Scope/1

== system suspension_controller_road_condition2/hybrid hook/rear_sum/Hybrid controller1 ==
  zc_dot : Inport
  zc_dot - zr_dot : Inport  Port=2
  -zr_dot*(zc_dot-zr_dot) : Inport  Port=3
  Add : Sum
  Constant : Constant  Value=2838
  Constant1 : Constant  Value=258
  Constant2 : Constant  Value=2838
  Constant3 : Constant  Value=258
  If : If  IfExpression=u1 >= 0  ZeroCross=off
  If Action Subsystem : Subsystem  TreatAsAtomicUnit=on
  If Action Subsystem1 : Subsystem  TreatAsAtomicUnit=on
  If Action Subsystem2 : Subsystem  TreatAsAtomicUnit=on
  If Action Subsystem3 : Subsystem  TreatAsAtomicUnit=on
  If1 : If  IfExpression=u1 >= 0  ZeroCross=off
  Merge : Merge
  Merge1 : Merge
  Product : Product
  Csa : Outport
  wires:
  zc_dot/1 -> Product/1
  Product/1 -> If/1
  If/1 -> If Action Subsystem/Action
  Constant/1 -> If Action Subsystem/1(In1)
  If/2 -> If Action Subsystem1/Action
  If Action Subsystem/1(Csa) -> Merge/1
  If Action Subsystem1/1(Out1) -> Merge/2
  Constant1/1 -> If Action Subsystem1/1(In1)
  zc_dot - zr_dot/1 -> Product/2
  If Action Subsystem2/1(Csa) -> Merge1/1
  If Action Subsystem3/1(Out1) -> Merge1/2
  If1/1 -> If Action Subsystem2/Action
  -zr_dot*(zc_dot-zr_dot)/1 -> If1/1
  Constant2/1 -> If Action Subsystem2/1(In1)
  Constant3/1 -> If Action Subsystem3/1(In1)
  If1/2 -> If Action Subsystem3/Action
  Merge/1 -> Add/1
  Merge1/1 -> Add/2
  Add/1 -> Csa/1

== system suspension_controller_road_condition2/hybrid hook/rear_sum/Road Condition2 ==
  Product : Product  Inputs=3
  Saturation : Saturate  LowerLimit=0
  Scope : Scope
  Signal Generator : SignalGenerator  Amplitude=0.15  Frequency=1.852
  Step : Step  SampleTime=1.08
  Step1 : Step  Before=1  After=0  SampleTime=4
  Output : Outport
  wires:
  Signal Generator/1 -> Product/1
  Step/1 -> Product/2
  Step1/1 -> Product/3
  Product/1 -> Output/1, Saturation/1
  Saturation/1 -> Scope/1

== system suspension_controller_road_condition2/passive/Front_sum/Road Condition2 ==
  Product : Product  Inputs=3
  Saturation : Saturate  LowerLimit=0
  Scope : Scope
  Signal Generator : SignalGenerator  Amplitude=0.15  Frequency=1.852
  Step : Step  SampleTime=1.08
  Step1 : Step  Before=1  After=0  SampleTime=4
  Output : Outport
  wires:
  Signal Generator/1 -> Product/1
  Step/1 -> Product/2
  Step1/1 -> Product/3
  Product/1 -> Output/1, Saturation/1
  Saturation/1 -> Scope/1

== system suspension_controller_road_condition2/passive/Rear_sum/Road Condition2 ==
  Product : Product  Inputs=3
  Saturation : Saturate  LowerLimit=0
  Scope : Scope
  Signal Generator : SignalGenerator  Amplitude=0.15  Frequency=1.852
  Step : Step  SampleTime=1.08
  Step1 : Step  Before=1  After=0  SampleTime=4
  Output : Outport
  wires:
  Signal Generator/1 -> Product/1
  Step/1 -> Product/2
  Step1/1 -> Product/3
  Product/1 -> Output/1, Saturation/1
  Saturation/1 -> Scope/1
